simulink model "lab8CTRLsim"  (R2021b)
settings: Solver=VariableStepAuto  StartTime=0.0  StopTime=6  RelTol=1e-3
undefined symbols (not defined in the file): A, B, k, r0, r1, r2, tao, tm
settings Model: Creator=nicol  LastModifiedBy=nicol

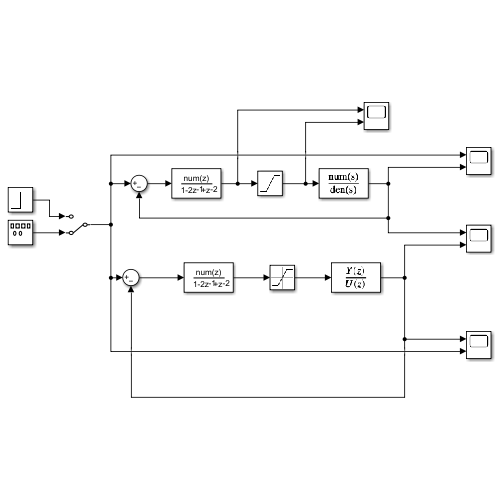
[thumbnail: Simulink's stored preview of the top-level diagram]
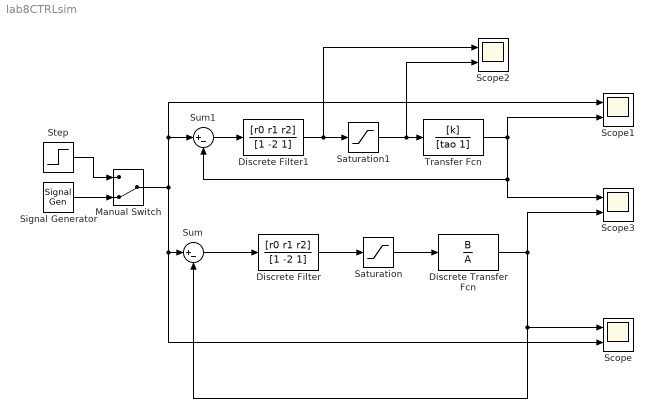
== system lab8CTRLsim ==
  Discrete Transfer Fcn : DiscreteTransferFcn  Numerator=B  Denominator=A  SampleTime=tm
  Discrete Filter : DiscreteFilter  Numerator=[r0 r1 r2]  Denominator=[1 -2 1]  SampleTime=tm
  Discrete Filter1 : DiscreteFilter  Numerator=[r0 r1 r2]  Denominator=[1 -2 1]  SampleTime=tm
  Manual Switch : ManualSwitch  CurrentSetting=0
  Saturation : Saturate  UpperLimit=8.2  LowerLimit=-8.2
  Saturation1 : Saturate  UpperLimit=8.2  LowerLimit=-8.2
  Scope{,1..3} (4 alike) : Scope  NumInputPorts=2
  Signal Generator : SignalGenerator
  Step : Step  Time=0  SampleTime=0
  Sum : Sum  Inputs=|+-
  Sum1 : Sum  Inputs=|+-
  Transfer Fcn : TransferFcn  Numerator=[k]  Denominator=[tao 1]
  wires:
  Discrete Filter/1 -> Saturation/1
  Sum/1 -> Discrete Filter/1
  Sum1/1 -> Discrete Filter1/1
  Saturation/1 -> Discrete Transfer Fcn/1
  Discrete Filter1/1 -> Scope2/1, Saturation1/1
  Saturation1/1 -> Scope2/2, Transfer Fcn/1
  Transfer Fcn/1 -> Scope3/1, Sum1/2, Scope1/2
  Discrete Transfer Fcn/1 -> Sum/2, Scope/1, Scope3/2
  Manual Switch/1 -> Scope/2, Sum/1, Scope1/1, Sum1/1
  Signal Generator/1 -> Manual Switch/2
  Step/1 -> Manual Switch/1
